simulink model "MOBATSim"  (R2020b)
settings: Solver=FixedStepAuto  StartTime=0.0  StopTime=Sim_t  FixedStep=0.01  MinStep=0.01  RelTol=1e-2
values from neighbouring files (symbols this model uses):
  maxSpeed = car.dynamics.maxSpeed    [VehiclePathPlanner.m]    (also in VehiclePathPlanner1.m; VehiclePathPlanner_AStar.m; VehiclePathPlanner_Astar.m; VehiclePathPlanner_DStarExtraLight.m)
  Vehicles = evalin('base','Vehicles')    [Infrastructure.m]    (also in VehicleSensors.m)
undefined symbols (not defined in the file or in its folder): default_spacing, delayTimeV3, FI_distance, FI_speed, max_ac, meters, min_ac, MinDeceleration, SafeDistance, Sim_Ts, time_gap, Ts, v_set, Vehicle_id, verr_gain, vx_gain, xerr_gain
libraries: simulink x43, pid_lib x15, drivingvehiclecontroller x11, robotmobilelib x11, autolibshared x4, robotalgslib x3, mpcadaslib x1
(part 2 of 7)

== system MOBATSim/Vehicle Model 6 ==
  note: Perception
  note: Decision-Making
  note: Control
  Behavioural Planner : MATLABSystem  System=VehicleDrivingMode  Vehicle_id=Vehicle_id  SimulateUsing=Interpreted execution
      mask Type: VehicleDrivingMode
      mask Display:
      | image('BehaviouralPlanner.png');
      | port_label('input',1,'LeaderSpeed');
      | port_label('input',2,'LeaderDistance');
      | port_label('input',3,'emergencyCase');
      | port_label('output',1,'SpeedReference');
      | port_label('output',2,'DistanceReference');
      | port_label('output',3,'LeadSpeed');
      | port_label('output',4,'DrivingMode');
      | port_label('output',5,'Dist2Stop');
      | port_label('output',6,'laneChange');
  Longitudinal and Lateral Controllers : Subsystem
  Safety Filter : Subsystem
  Transform to MOBATSim Coordinates : Subsystem
  Vehicle Model - Kinematic 3DOF Single Track : Subsystem  mask{Vehicle_id=Vehicle_id}
      mask prompts: Vehicle_id "Vehicle ID"
  Vehicle Path Planner : MATLABSystem  System=VehiclePathPlanner_Astar  Vehicle_id=Vehicle_id  SimulateUsing=Interpreted execution
      mask Type: VehiclePathPlanner_Astar
      mask Display:
      | image('PathPlanner.png');
      | port_label('input',1,'CommunicationIDs');
      | port_label('output',1,'waypointReached');
  Vehicle Sensors : MATLABSystem  System=VehicleSensors  Vehicle_id=Vehicle_id  Tsample=Sim_Ts  OffsetTime=0  SimulateUsing=Interpreted execution
      mask Type: VehicleSensors
      mask Display:
      | image('sensor.png');
      | port_label('output',1,'V2VcommIDs');
      | port_label('output',2,'distanceToLeading');
  Vehicle Situation Awareness : MATLABSystem  System=VehicleSituationAwareness  Vehicle_id=Vehicle_id  SimulateUsing=Interpreted execution
      mask Type: VehicleSituationAwareness
      mask Display:
      | image('situationAwareness.png');
      | port_label('input',1,'detectionFrontSensor');
      | port_label('output',1,'leaderSpeed');
      | port_label('output',2,'leaderDistance');
      | port_label('output',3,'emergencyCase');
  Vehicle V2I Output : MATLABSystem  System=VehicleV2I_Out  Vehicle_id=Vehicle_id  SimulateUsing=Interpreted execution
      mask Type: VehicleV2I_Out
      mask Display:
      | image('V2I.png');
      | port_label('input',1,'waypointReached');
      | port_label('output',1,'V2Idata');
  Position : Outport  VectorParamsAs1DForOutWhenUnconnected=off
  Orientation : Outport  Port=2  VectorParamsAs1DForOutWhenUnconnected=off
  Speed : Outport  Port=3  VectorParamsAs1DForOutWhenUnconnected=off
  V_Network_Out : Outport  Port=4  VectorParamsAs1DForOutWhenUnconnected=off
  wires:
  Vehicle Sensors/2 -> Vehicle Situation Awareness/1
  Vehicle Situation Awareness/1 -> Behavioural Planner/1
  Vehicle Path Planner/1 -> Vehicle V2I Output/1
  Vehicle Sensors/1 -> Vehicle Path Planner/1
  Vehicle V2I Output/1 -> V_Network_Out/1
  Vehicle Situation Awareness/3 -> Behavioural Planner/3
  Vehicle Situation Awareness/2 -> Behavioural Planner/2
  Behavioural Planner/1 -> Longitudinal and Lateral Controllers/1(Speed Reference)
  Behavioural Planner/2 -> Longitudinal and Lateral Controllers/2(Inter Vehicular Distance)
  Behavioural Planner/3 -> Longitudinal and Lateral Controllers/3(Lead Speed)
  Behavioural Planner/4 -> Longitudinal and Lateral Controllers/4(drivingMode)
  Behavioural Planner/5 -> Longitudinal and Lateral Controllers/5(Dist2Stop)
  Transform to MOBATSim Coordinates/1(Position) -> Position/1
  Transform to MOBATSim Coordinates/2(Orientation) -> Orientation/1
  Vehicle Model - Kinematic 3DOF Single Track/2(xdot) -> Longitudinal and Lateral Controllers/7(Actual Speed), Speed/1
  Vehicle Model - Kinematic 3DOF Single Track/1(Pose) -> Longitudinal and Lateral Controllers/8(Actual Pose), Transform to MOBATSim Coordinates/1(Pose)
  Longitudinal and Lateral Controllers/1(ref Acc) -> Safety Filter/1(Reference Acceleration)
  Longitudinal and Lateral Controllers/2(ref Steering) -> Safety Filter/2(Reference Steering Angle)
  Safety Filter/1(Steering Angle Cmd) -> Vehicle Model - Kinematic 3DOF Single Track/1(WhlAngF)
  Safety Filter/2(Speed_input) -> Vehicle Model - Kinematic 3DOF Single Track/2(xdotin)
  Behavioural Planner/6 -> Longitudinal and Lateral Controllers/6(laneChange)

== system MOBATSim/Vehicle Model 7 ==
  note: Perception
  note: Decision-Making
  note: Control
  Behavioural Planner : MATLABSystem  System=VehicleDrivingMode  Vehicle_id=Vehicle_id  SimulateUsing=Interpreted execution
      mask Type: VehicleDrivingMode
      mask Display:
      | image('BehaviouralPlanner.png');
      | port_label('input',1,'LeaderSpeed');
      | port_label('input',2,'LeaderDistance');
      | port_label('input',3,'emergencyCase');
      | port_label('output',1,'SpeedReference');
      | port_label('output',2,'DistanceReference');
      | port_label('output',3,'LeadSpeed');
      | port_label('output',4,'DrivingMode');
      | port_label('output',5,'Dist2Stop');
      | port_label('output',6,'laneChange');
  Longitudinal and Lateral Controllers : Subsystem
  Safety Filter : Subsystem
  Transform to MOBATSim Coordinates : Subsystem
  Vehicle Model - Kinematic 3DOF Single Track : Subsystem  mask{Vehicle_id=Vehicle_id}
      mask prompts: Vehicle_id "Vehicle ID"
  Vehicle Path Planner : MATLABSystem  System=VehiclePathPlanner_Astar  Vehicle_id=Vehicle_id  SimulateUsing=Interpreted execution
      mask Type: VehiclePathPlanner_Astar
      mask Display:
      | image('PathPlanner.png');
      | port_label('input',1,'CommunicationIDs');
      | port_label('output',1,'waypointReached');
  Vehicle Sensors : MATLABSystem  System=VehicleSensors  Vehicle_id=Vehicle_id  Tsample=Sim_Ts  OffsetTime=0  SimulateUsing=Interpreted execution
      mask Type: VehicleSensors
      mask Display:
      | image('sensor.png');
      | port_label('output',1,'V2VcommIDs');
      | port_label('output',2,'distanceToLeading');
  Vehicle Situation Awareness : MATLABSystem  System=VehicleSituationAwareness  Vehicle_id=Vehicle_id  SimulateUsing=Interpreted execution
      mask Type: VehicleSituationAwareness
      mask Display:
      | image('situationAwareness.png');
      | port_label('input',1,'detectionFrontSensor');
      | port_label('output',1,'leaderSpeed');
      | port_label('output',2,'leaderDistance');
      | port_label('output',3,'emergencyCase');
  Vehicle V2I Output : MATLABSystem  System=VehicleV2I_Out  Vehicle_id=Vehicle_id  SimulateUsing=Interpreted execution
      mask Type: VehicleV2I_Out
      mask Display:
      | image('V2I.png');
      | port_label('input',1,'waypointReached');
      | port_label('output',1,'V2Idata');
  Position : Outport  VectorParamsAs1DForOutWhenUnconnected=off
  Orientation : Outport  Port=2  VectorParamsAs1DForOutWhenUnconnected=off
  Speed : Outport  Port=3  VectorParamsAs1DForOutWhenUnconnected=off
  V_Network_Out : Outport  Port=4  VectorParamsAs1DForOutWhenUnconnected=off
  wires:
  Vehicle Sensors/2 -> Vehicle Situation Awareness/1
  Vehicle Situation Awareness/1 -> Behavioural Planner/1
  Vehicle Path Planner/1 -> Vehicle V2I Output/1
  Vehicle Sensors/1 -> Vehicle Path Planner/1
  Vehicle V2I Output/1 -> V_Network_Out/1
  Vehicle Situation Awareness/3 -> Behavioural Planner/3
  Vehicle Situation Awareness/2 -> Behavioural Planner/2
  Behavioural Planner/1 -> Longitudinal and Lateral Controllers/1(Speed Reference)
  Behavioural Planner/2 -> Longitudinal and Lateral Controllers/2(Inter Vehicular Distance)
  Behavioural Planner/3 -> Longitudinal and Lateral Controllers/3(Lead Speed)
  Behavioural Planner/4 -> Longitudinal and Lateral Controllers/4(drivingMode)
  Behavioural Planner/5 -> Longitudinal and Lateral Controllers/5(Dist2Stop)
  Transform to MOBATSim Coordinates/1(Position) -> Position/1
  Transform to MOBATSim Coordinates/2(Orientation) -> Orientation/1
  Vehicle Model - Kinematic 3DOF Single Track/2(xdot) -> Longitudinal and Lateral Controllers/7(Actual Speed), Speed/1
  Vehicle Model - Kinematic 3DOF Single Track/1(Pose) -> Longitudinal and Lateral Controllers/8(Actual Pose), Transform to MOBATSim Coordinates/1(Pose)
  Longitudinal and Lateral Controllers/1(ref Acc) -> Safety Filter/1(Reference Acceleration)
  Longitudinal and Lateral Controllers/2(ref Steering) -> Safety Filter/2(Reference Steering Angle)
  Safety Filter/1(Steering Angle Cmd) -> Vehicle Model - Kinematic 3DOF Single Track/1(WhlAngF)
  Safety Filter/2(Speed_input) -> Vehicle Model - Kinematic 3DOF Single Track/2(xdotin)
  Behavioural Planner/6 -> Longitudinal and Lateral Controllers/6(laneChange)

== system MOBATSim/Vehicle Model 8 ==
  note: Perception
  note: Decision-Making
  note: Control
  Behavioural Planner : MATLABSystem  System=VehicleDrivingMode  Vehicle_id=Vehicle_id  SimulateUsing=Interpreted execution
      mask Type: VehicleDrivingMode
      mask Display:
      | image('BehaviouralPlanner.png');
      | port_label('input',1,'LeaderSpeed');
      | port_label('input',2,'LeaderDistance');
      | port_label('input',3,'emergencyCase');
      | port_label('output',1,'SpeedReference');
      | port_label('output',2,'DistanceReference');
      | port_label('output',3,'LeadSpeed');
      | port_label('output',4,'DrivingMode');
      | port_label('output',5,'Dist2Stop');
      | port_label('output',6,'laneChange');
  Longitudinal and Lateral Controllers : Subsystem
  Safety Filter : Subsystem
  Transform to MOBATSim Coordinates : Subsystem
  Vehicle Model - Kinematic 3DOF Single Track : Subsystem  mask{Vehicle_id=Vehicle_id}
      mask prompts: Vehicle_id "Vehicle ID"
  Vehicle Path Planner : MATLABSystem  System=VehiclePathPlanner_Astar  Vehicle_id=Vehicle_id  SimulateUsing=Interpreted execution
      mask Type: VehiclePathPlanner_Astar
      mask Display:
      | image('PathPlanner.png');
      | port_label('input',1,'CommunicationIDs');
      | port_label('output',1,'waypointReached');
  Vehicle Sensors : MATLABSystem  System=VehicleSensors  Vehicle_id=Vehicle_id  Tsample=Sim_Ts  OffsetTime=0  SimulateUsing=Interpreted execution
      mask Type: VehicleSensors
      mask Display:
      | image('sensor.png');
      | port_label('output',1,'V2VcommIDs');
      | port_label('output',2,'distanceToLeading');
  Vehicle Situation Awareness : MATLABSystem  System=VehicleSituationAwareness  Vehicle_id=Vehicle_id  SimulateUsing=Interpreted execution
      mask Type: VehicleSituationAwareness
      mask Display:
      | image('situationAwareness.png');
      | port_label('input',1,'detectionFrontSensor');
      | port_label('output',1,'leaderSpeed');
      | port_label('output',2,'leaderDistance');
      | port_label('output',3,'emergencyCase');
  Vehicle V2I Output : MATLABSystem  System=VehicleV2I_Out  Vehicle_id=Vehicle_id  SimulateUsing=Interpreted execution
      mask Type: VehicleV2I_Out
      mask Display:
      | image('V2I.png');
      | port_label('input',1,'waypointReached');
      | port_label('output',1,'V2Idata');
  Position : Outport  VectorParamsAs1DForOutWhenUnconnected=off
  Orientation : Outport  Port=2  VectorParamsAs1DForOutWhenUnconnected=off
  Speed : Outport  Port=3  VectorParamsAs1DForOutWhenUnconnected=off
  V_Network_Out : Outport  Port=4  VectorParamsAs1DForOutWhenUnconnected=off
  wires:
  Vehicle Sensors/2 -> Vehicle Situation Awareness/1
  Vehicle Situation Awareness/1 -> Behavioural Planner/1
  Vehicle Path Planner/1 -> Vehicle V2I Output/1
  Vehicle Sensors/1 -> Vehicle Path Planner/1
  Vehicle V2I Output/1 -> V_Network_Out/1
  Vehicle Situation Awareness/3 -> Behavioural Planner/3
  Vehicle Situation Awareness/2 -> Behavioural Planner/2
  Behavioural Planner/1 -> Longitudinal and Lateral Controllers/1(Speed Reference)
  Behavioural Planner/2 -> Longitudinal and Lateral Controllers/2(Inter Vehicular Distance)
  Behavioural Planner/3 -> Longitudinal and Lateral Controllers/3(Lead Speed)
  Behavioural Planner/4 -> Longitudinal and Lateral Controllers/4(drivingMode)
  Behavioural Planner/5 -> Longitudinal and Lateral Controllers/5(Dist2Stop)
  Transform to MOBATSim Coordinates/1(Position) -> Position/1
  Transform to MOBATSim Coordinates/2(Orientation) -> Orientation/1
  Vehicle Model - Kinematic 3DOF Single Track/2(xdot) -> Longitudinal and Lateral Controllers/7(Actual Speed), Speed/1
  Vehicle Model - Kinematic 3DOF Single Track/1(Pose) -> Longitudinal and Lateral Controllers/8(Actual Pose), Transform to MOBATSim Coordinates/1(Pose)
  Longitudinal and Lateral Controllers/1(ref Acc) -> Safety Filter/1(Reference Acceleration)
  Longitudinal and Lateral Controllers/2(ref Steering) -> Safety Filter/2(Reference Steering Angle)
  Safety Filter/1(Steering Angle Cmd) -> Vehicle Model - Kinematic 3DOF Single Track/1(WhlAngF)
  Safety Filter/2(Speed_input) -> Vehicle Model - Kinematic 3DOF Single Track/2(xdotin)
  Behavioural Planner/6 -> Longitudinal and Lateral Controllers/6(laneChange)

== system MOBATSim/Vehicle Model 9 ==
  note: Perception
  note: Decision-Making
  note: Control
  Behavioural Planner : MATLABSystem  System=VehicleDrivingMode  Vehicle_id=Vehicle_id  SimulateUsing=Interpreted execution
      mask Type: VehicleDrivingMode
      mask Display:
      | image('BehaviouralPlanner.png');
      | port_label('input',1,'LeaderSpeed');
      | port_label('input',2,'LeaderDistance');
      | port_label('input',3,'emergencyCase');
      | port_label('output',1,'SpeedReference');
      | port_label('output',2,'DistanceReference');
      | port_label('output',3,'LeadSpeed');
      | port_label('output',4,'DrivingMode');
      | port_label('output',5,'Dist2Stop');
      | port_label('output',6,'laneChange');
  Longitudinal and Lateral Controllers : Subsystem
  Safety Filter : Subsystem
  Transform to MOBATSim Coordinates : Subsystem
  Vehicle Model - Kinematic 3DOF Single Track : Subsystem  mask{Vehicle_id=Vehicle_id}
      mask prompts: Vehicle_id "Vehicle ID"
  Vehicle Path Planner : MATLABSystem  System=VehiclePathPlanner_Astar  Vehicle_id=Vehicle_id  SimulateUsing=Interpreted execution
      mask Type: VehiclePathPlanner_Astar
      mask Display:
      | image('PathPlanner.png');
      | port_label('input',1,'CommunicationIDs');
      | port_label('output',1,'waypointReached');
  Vehicle Sensors : MATLABSystem  System=VehicleSensors  Vehicle_id=Vehicle_id  Tsample=Sim_Ts  OffsetTime=0  SimulateUsing=Interpreted execution
      mask Type: VehicleSensors
      mask Display:
      | image('sensor.png');
      | port_label('output',1,'V2VcommIDs');
      | port_label('output',2,'distanceToLeading');
  Vehicle Situation Awareness : MATLABSystem  System=VehicleSituationAwareness  Vehicle_id=Vehicle_id  SimulateUsing=Interpreted execution
      mask Type: VehicleSituationAwareness
      mask Display:
      | image('situationAwareness.png');
      | port_label('input',1,'detectionFrontSensor');
      | port_label('output',1,'leaderSpeed');
      | port_label('output',2,'leaderDistance');
      | port_label('output',3,'emergencyCase');
  Vehicle V2I Output : MATLABSystem  System=VehicleV2I_Out  Vehicle_id=Vehicle_id  SimulateUsing=Interpreted execution
      mask Type: VehicleV2I_Out
      mask Display:
      | image('V2I.png');
      | port_label('input',1,'waypointReached');
      | port_label('output',1,'V2Idata');
  Position : Outport  VectorParamsAs1DForOutWhenUnconnected=off
  Orientation : Outport  Port=2  VectorParamsAs1DForOutWhenUnconnected=off
  Speed : Outport  Port=3  VectorParamsAs1DForOutWhenUnconnected=off
  V_Network_Out : Outport  Port=4  VectorParamsAs1DForOutWhenUnconnected=off
  wires:
  Vehicle Sensors/2 -> Vehicle Situation Awareness/1
  Vehicle Situation Awareness/1 -> Behavioural Planner/1
  Vehicle Path Planner/1 -> Vehicle V2I Output/1
  Vehicle Sensors/1 -> Vehicle Path Planner/1
  Vehicle V2I Output/1 -> V_Network_Out/1
  Vehicle Situation Awareness/3 -> Behavioural Planner/3
  Vehicle Situation Awareness/2 -> Behavioural Planner/2
  Behavioural Planner/1 -> Longitudinal and Lateral Controllers/1(Speed Reference)
  Behavioural Planner/2 -> Longitudinal and Lateral Controllers/2(Inter Vehicular Distance)
  Behavioural Planner/3 -> Longitudinal and Lateral Controllers/3(Lead Speed)
  Behavioural Planner/4 -> Longitudinal and Lateral Controllers/4(drivingMode)
  Behavioural Planner/5 -> Longitudinal and Lateral Controllers/5(Dist2Stop)
  Transform to MOBATSim Coordinates/1(Position) -> Position/1
  Transform to MOBATSim Coordinates/2(Orientation) -> Orientation/1
  Vehicle Model - Kinematic 3DOF Single Track/2(xdot) -> Longitudinal and Lateral Controllers/7(Actual Speed), Speed/1
  Vehicle Model - Kinematic 3DOF Single Track/1(Pose) -> Longitudinal and Lateral Controllers/8(Actual Pose), Transform to MOBATSim Coordinates/1(Pose)
  Longitudinal and Lateral Controllers/1(ref Acc) -> Safety Filter/1(Reference Acceleration)
  Longitudinal and Lateral Controllers/2(ref Steering) -> Safety Filter/2(Reference Steering Angle)
  Safety Filter/1(Steering Angle Cmd) -> Vehicle Model - Kinematic 3DOF Single Track/1(WhlAngF)
  Safety Filter/2(Speed_input) -> Vehicle Model - Kinematic 3DOF Single Track/2(xdotin)
  Behavioural Planner/6 -> Longitudinal and Lateral Controllers/6(laneChange)

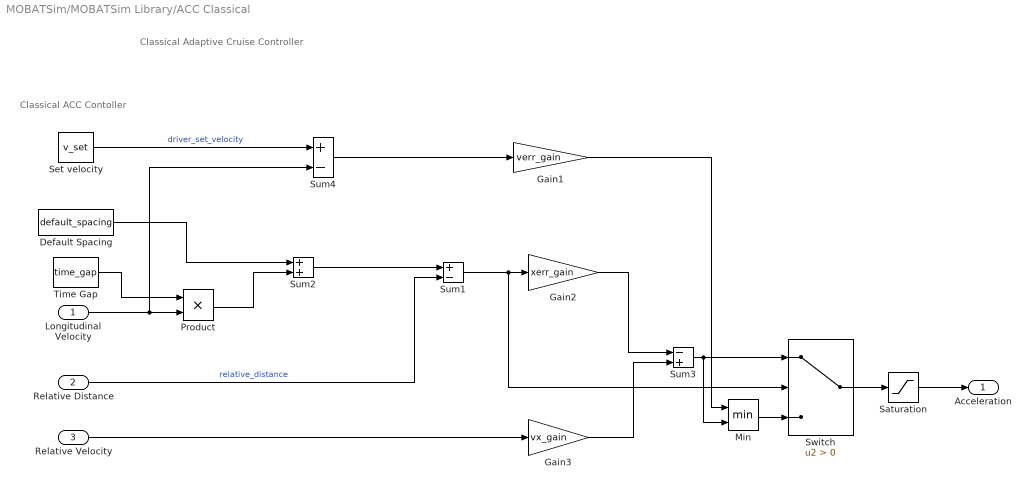
== system MOBATSim/MOBATSim Library/ACC Classical ==
  note: Classical ACC Contoller
  note: Classical Adaptive Cruise Controller
  Longitudinal Velocity : Inport
  Relative Distance : Inport  Port=2
  Relative Velocity : Inport  Port=3
  Default Spacing : Constant  Value=default_spacing  SampleTime=Ts
  Gain1 : Gain  Gain=verr_gain
  Gain2 : Gain  Gain=xerr_gain
  Gain3 : Gain  Gain=vx_gain
  Min : MinMax  Inputs=2
  Product : Product
  Saturation : Saturate  UpperLimit=max_ac  LowerLimit=min_ac
  Set velocity : Constant  Value=v_set  SampleTime=Ts
  Sum1 : Sum  Inputs=+-
  Sum2 : Sum
  Sum3 : Sum  Inputs=-+
  Sum4 : Sum  Inputs=+-
  Switch : Switch  Criteria=u2 > Threshold
  Time Gap : Constant  Value=time_gap  SampleTime=Ts
  Acceleration : Outport  VectorParamsAs1DForOutWhenUnconnected=off
  wires:
  Longitudinal Velocity/1 -> Product/2, Sum4/2
  Default Spacing/1 -> Sum2/1
  Gain2/1 -> Sum3/1
  Sum4/1 -> Gain1/1
  Min/1 -> Switch/3
  Gain3/1 -> Sum3/2
  Switch/1 -> Saturation/1
  Relative Velocity/1 -> Gain3/1
  Time Gap/1 -> Product/1
  Saturation/1 -> Acceleration/1
  Product/1 -> Sum2/2
  Set velocity/1 -> Sum4/1  "driver_set_velocity"
  Sum3/1 -> Min/2, Switch/1
  Sum1/1 -> Switch/2, Gain2/1
  Gain1/1 -> Min/1
  Relative Distance/1 -> Sum1/2  "relative_distance"
  Sum2/1 -> Sum1/1

== system MOBATSim/MOBATSim Library/Old Vehicle 3 Dynamic Bicycle Model with Pure Pursuit ==
  Speed Reference : Inport
  Inter Vehicular Distance : Inport  Port=2
  Lead Speed : Inport  Port=3
  drivingMode : Inport  Port=4
  CollisionStatus : Inport  Port=5
  Dist2Stop : Inport  Port=6
  Longitudinal Speed Control : Subsystem
  Reference Waypoint Generation : Subsystem
  Vehicle Dynamics Interface : Subsystem
  Vehicle Kinematic 3DOF Single Track : Subsystem  mask{Vehicle_id=Vehicle_id}
      mask prompts: Vehicle_id "Vehicle ID"
  X : Outport
  Y : Outport  Port=2
  yaw : Outport  Port=3
  wires:
  Reference Waypoint Generation/1(Target Direction) -> Vehicle Dynamics Interface/3(Target Direction)
  Vehicle Kinematic 3DOF Single Track/4(xdot) -> Longitudinal Speed Control/6(Actual Speed), Reference Waypoint Generation/4(Speed)
  Lead Speed/1 -> Longitudinal Speed Control/3(Lead Speed)
  Vehicle Dynamics Interface/1(Actual Steering Angle) -> Vehicle Kinematic 3DOF Single Track/1(WhlAngF)
  CollisionStatus/1 -> Vehicle Dynamics Interface/2(CollisionStatus)
  Vehicle Kinematic 3DOF Single Track/1(X) -> X/1, Reference Waypoint Generation/1(Xpos)
  Dist2Stop/1 -> Longitudinal Speed Control/5(Dist2Stop)
  Vehicle Dynamics Interface/2(Actual Speed) -> Vehicle Kinematic 3DOF Single Track/2(xdotin)
  drivingMode/1 -> Longitudinal Speed Control/4(Driving Mode), Reference Waypoint Generation/5(drivingMode)
  Vehicle Kinematic 3DOF Single Track/2(Y) -> Y/1, Reference Waypoint Generation/2(Ypos)
  Vehicle Kinematic 3DOF Single Track/3(yaw) -> yaw/1, Reference Waypoint Generation/3(Psi)
  Longitudinal Speed Control/1(Longitduinal Acceleration Command) -> Vehicle Dynamics Interface/1(Acceleration)
  Speed Reference/1 -> Longitudinal Speed Control/1(Speed Reference)
  Inter Vehicular Distance/1 -> Longitudinal Speed Control/2(Inter Vehicular Distance)

== system MOBATSim/MOBATSim Library/Old Vehicle 5 Dual Track ==
  Speed Reference : Inport
  Inter Vehicular Distance : Inport  Port=2
  Lead Speed : Inport  Port=3
  drivingMode : Inport  Port=4
  CollisionStatus : Inport  Port=5
  Dist2Stop : Inport  Port=6
  Longitudinal Speed Control : Subsystem
  Reference Waypoint Generation : Subsystem
  Vehicle Dynamics Interface : Subsystem
  Vehicle Kinematic 3DOF Single Track : Subsystem  mask{Vehicle_id=Vehicle_id}
      mask prompts: Vehicle_id "Vehicle ID"
  X : Outport
  Y : Outport  Port=2
  yaw : Outport  Port=3
  wires:
  Vehicle Kinematic 3DOF Single Track/1(X) -> X/1, Reference Waypoint Generation/1(Xpos)
  Reference Waypoint Generation/1(SteerCmd_Stanley) -> Vehicle Dynamics Interface/3(SteerCmd_Stanley)
  Vehicle Dynamics Interface/2(Actual Speed) -> Vehicle Kinematic 3DOF Single Track/2(xdotin)
  Vehicle Kinematic 3DOF Single Track/2(Y) -> Y/1, Reference Waypoint Generation/2(Ypos)
  Vehicle Kinematic 3DOF Single Track/4(xdot) -> Longitudinal Speed Control/6(Actual Speed), Reference Waypoint Generation/4(Speed)
  drivingMode/1 -> Reference Waypoint Generation/5(drivingMode), Longitudinal Speed Control/4(Driving Mode)
  Vehicle Dynamics Interface/1(Actual Steering Angle) -> Vehicle Kinematic 3DOF Single Track/1(WhlAngF)
  Vehicle Kinematic 3DOF Single Track/3(yaw) -> yaw/1, Reference Waypoint Generation/3(Psi)
  Longitudinal Speed Control/1(Longitduinal Acceleration Command) -> Vehicle Dynamics Interface/1(Acceleration)
  Dist2Stop/1 -> Longitudinal Speed Control/5(Dist2Stop)
  CollisionStatus/1 -> Vehicle Dynamics Interface/2(CollisionStatus)
  Inter Vehicular Distance/1 -> Longitudinal Speed Control/2(Inter Vehicular Distance)
  Lead Speed/1 -> Longitudinal Speed Control/3(Lead Speed)
  Speed Reference/1 -> Longitudinal Speed Control/1(Speed Reference)

== system MOBATSim/MOBATSim Library/Platoon Controller - PID ==
  Inter Vehicular Distance : Inport
  Lead Speed : Inport  Port=2
  Vehicle Speed : Inport  Port=3
  Compare To Constant : simulink/Logic and Bit Operations/Compare To Constant  relop=>  const=2  OutDataTypeStr=uint8
  Constant : Constant  Value=meters
  Gain : Gain  Gain=1.4
  Multiport Switch : MultiPortSwitch  DataPortOrder=Zero-based contiguous  Inputs=2  zeroidx=on
  PID Controller5 : pid_lib/PID Controller  Controller=PID  Form=Parallel  TimeDomain=Continuous-time  UseExternalTs=off  SampleTime=-1  IntegratorMethod=Forward Euler  FilterMethod=Forward Euler  ControllerParametersSource=internal  P=2.0341199375219  I=0.0356576460366845  D=2.08363010404189  UseFilter=on  N=233.214579742572  TunerSelectOption=Transfer Function Based (PID Tuner App)  InitialConditionSource=internal  InitialConditionForIntegrator=0  InitialConditionForFilter=0  DifferentiatorICPrevScaledInput=0  ExternalReset=none  TrackingMode=off  Kt=1  LimitOutput=on  SatLimitsSource=internal  UpperSaturationLimit=100  LowerSaturationLimit=-100  LinearizeAsGain=on  AntiWindupMode=clamping  Kb=1  POutMin=[]  POutMax=[]  IOutMin=[]  IOutMax=[]  DOutMin=[]  DOutMax=[]  NOutMin=[]  NOutMax=[]  SumOutMin=[]  SumOutMax=[]  SaturationOutMin=[]  SaturationOutMax=[]  PParamMin=[]  PParamMax=[]  IParamMin=[]  IParamMax=[]  DParamMin=[]  DParamMax=[]  NParamMin=[]  NParamMax=[]  KbParamMin=[]  KbParamMax=[]  KtParamMin=[]  KtParamMax=[]  KbOutMin=[]  KbOutMax=[]  KtOutMin=[]  KtOutMax=[]  IntegratorOutMin=[]  IntegratorOutMax=[]  FilterOutMin=[]  FilterOutMax=[]  SumI1OutMin=[]  SumI1OutMax=[]  SumI2OutMin=[]  SumI2OutMax=[]  SumI3OutMin=[]  SumI3OutMax=[]  SumI4OutMin=[]  SumI4OutMax=[]  SumDOutMin=[]  SumDOutMax=[]  DifferentiatorOutMin=[]  DifferentiatorOutMax=[]  FilterDiffOutCoefMin=[]  FilterDiffOutCoefMax=[]  ReciprocalOutMin=[]  ReciprocalOutMax=[]  SumDenOutMin=[]  SumDenOutMax=[]  SumNumOutMin=[]  SumNumOutMax=[]  DivideOutMin=[]  DivideOutMax=[]  UdiffTsProdOutMin=[]  UdiffTsProdOutMax=[]  NTsProdOutMin=[]  NTsProdOutMax=[]  UintegralTsProdOutMin=[]  UintegralTsProdOutMax=[]  UngainTsProdOutMin=[]  UngainTsProdOutMax=[]  IntegratorContinuousStateAttributes=''  IntegratorStateMustResolveToSignalObject=off  IntegratorRTWStateStorageClass=Auto  FilterContinuousStateAttributes=''  FilterStateMustResolveToSignalObject=off  FilterRTWStateStorageClass=Auto  ParallelPVariant=InternalParameters  IdealPVariant=Disabled  IVariant=InternalParameters  DVariant=InternalParameters  IntegratorVariant=Continuous  SatVariant=Enabled  AWVariant=ContClampingParallel  PCopyVariant=Disabled  TRVariant=Disabled  FdbkBlocksVariant=Forward  IdealPFdbkVariant=Disabled  SatFdbkVariant=Disabled  DerivativeFilterVariant=ContFilter  NVariant=InternalParameters  NCopyVariant=Disabled  FilterICVariant=InternalICsFilter  IntegratorICVariant=InternalICs  ExternalResetVariant=Disabled  TRSumVariant=Passthrough  SumFdbkVariant=Disabled  SumVariant=Sum_PID  TsampFilterVariant=InternalTs  TsampNgainVariant=Passthrough  TsampIntegralVariant=Passthrough  ExternalSaturationOutDataTypeStr=Inherit: Same as second input
  Sum : Sum  Inputs=|-+
  Sum1 : Sum  Inputs=|++
  Sum2 : Sum  Inputs=|+-
  Transfer Fcn : TransferFcn  Numerator=[0.05]  Denominator=[1 2]
  ref speed : Outport  VectorParamsAs1DForOutWhenUnconnected=off
  wires:
  Transfer Fcn/1 -> PID Controller5/1
  Vehicle Speed/1 -> Gain/1, Sum/1
  PID Controller5/1 -> Multiport Switch/2
  Sum/1 -> Compare To Constant/1
  Multiport Switch/1 -> ref speed/1
  Compare To Constant/1 -> Multiport Switch/1
  Lead Speed/1 -> Sum/2, Multiport Switch/3
  Constant/1 -> Sum1/1
  Sum1/1 -> Sum2/2
  Gain/1 -> Sum1/2
  Sum2/1 -> Transfer Fcn/1
  Inter Vehicular Distance/1 -> Sum2/1

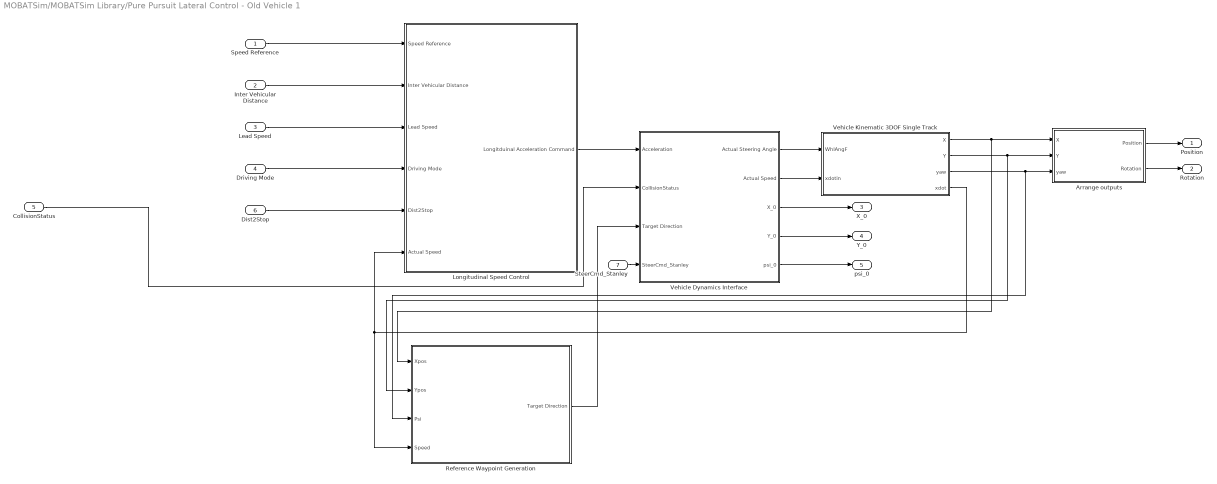
== system MOBATSim/MOBATSim Library/Pure Pursuit Lateral Control - Old Vehicle 1 ==
  Speed Reference : Inport
  Inter Vehicular Distance : Inport  Port=2
  Lead Speed : Inport  Port=3
  Driving Mode : Inport  Port=4
  CollisionStatus : Inport  Port=5
  Dist2Stop : Inport  Port=6
  SteerCmd_Stanley : Inport  Port=7
  Arrange outputs : Subsystem
  Longitudinal Speed Control : Subsystem
  Reference Waypoint Generation : Subsystem
  Vehicle Dynamics Interface : Subsystem
  Vehicle Kinematic 3DOF Single Track : Subsystem  mask{Vehicle_id=Vehicle_id}
      mask prompts: Vehicle_id "Vehicle ID"
  Position : Outport
  Rotation : Outport  Port=2
  X_0 : Outport  Port=3
  Y_0 : Outport  Port=4
  psi_0 : Outport  Port=5
  wires:
  Reference Waypoint Generation/1(Target Direction) -> Vehicle Dynamics Interface/3(Target Direction)
  Vehicle Kinematic 3DOF Single Track/1(X) -> Reference Waypoint Generation/1(Xpos), Arrange outputs/1(X)
  Vehicle Kinematic 3DOF Single Track/4(xdot) -> Longitudinal Speed Control/6(Actual Speed), Reference Waypoint Generation/4(Speed)
  SteerCmd_Stanley/1 -> Vehicle Dynamics Interface/4(SteerCmd_Stanley)
  Vehicle Dynamics Interface/2(Actual Speed) -> Vehicle Kinematic 3DOF Single Track/2(xdotin)
  Vehicle Dynamics Interface/1(Actual Steering Angle) -> Vehicle Kinematic 3DOF Single Track/1(WhlAngF)
  Vehicle Kinematic 3DOF Single Track/3(yaw) -> Reference Waypoint Generation/3(Psi), Arrange outputs/3(yaw)
  Longitudinal Speed Control/1(Longitduinal Acceleration Command) -> Vehicle Dynamics Interface/1(Acceleration)
  Vehicle Kinematic 3DOF Single Track/2(Y) -> Arrange outputs/2(Y), Reference Waypoint Generation/2(Ypos)
  Arrange outputs/1(Position) -> Position/1
  Inter Vehicular Distance/1 -> Longitudinal Speed Control/2(Inter Vehicular Distance)
  Driving Mode/1 -> Longitudinal Speed Control/4(Driving Mode)
  Dist2Stop/1 -> Longitudinal Speed Control/5(Dist2Stop)
  Lead Speed/1 -> Longitudinal Speed Control/3(Lead Speed)
  Speed Reference/1 -> Longitudinal Speed Control/1(Speed Reference)
  CollisionStatus/1 -> Vehicle Dynamics Interface/2(CollisionStatus)
  Vehicle Dynamics Interface/4(Y_0) -> Y_0/1
  Vehicle Dynamics Interface/3(X_0) -> X_0/1
  Arrange outputs/2(Rotation) -> Rotation/1
  Vehicle Dynamics Interface/5(psi_0) -> psi_0/1

== system MOBATSim/MOBATSim Library/Vehicle Model 5x ==
  note: Trajectory Planner
  note: Perception
  note: Decision Making
  Arrange outputs : Subsystem
  Behavioural Planner : MATLABSystem  System=VehicleDrivingMode  Vehicle_id=Vehicle_id  SimulateUsing=Interpreted execution
      mask Type: VehicleDrivingMode
      mask Display:
      | image('BehaviouralPlanner.png');
      | port_label('input',1,'LeaderSpeed');
      | port_label('input',2,'LeaderDistance');
      | port_label('input',3,'emergencyCase');
      | port_label('output',1,'SpeedReference');
      | port_label('output',2,'DistanceReference');
      | port_label('output',3,'LeadSpeed');
      | port_label('output',4,'DrivingMode');
      | port_label('output',5,'Dist2Stop');
  Old Vehicle 5 Dual Track : Subsystem
  Vehicle Path Planner : MATLABSystem  System=VehiclePathPlanner_Astar  Vehicle_id=Vehicle_id  SimulateUsing=Interpreted execution
      mask Type: VehiclePathPlanner_Astar
      mask Display:
      | image('PathPlanner.png');
      | port_label('input',1,'CommunicationIDs');
      | port_label('output',1,'waypointReached');
  Vehicle Sensors : MATLABSystem  System=VehicleSensors  Vehicle_id=Vehicle_id  Tsample=Sim_Ts  OffsetTime=0  SimulateUsing=Interpreted execution
      mask Type: VehicleSensors
      mask Display:
      | image('sensor.png');
      | port_label('output',1,'V2VcommIDs');
      | port_label('output',2,'distanceToLeading');
  Vehicle Situation Awareness : MATLABSystem  System=VehicleSituationAwareness  Vehicle_id=Vehicle_id  SimulateUsing=Interpreted execution
      mask Type: VehicleSituationAwareness
      mask Display:
      | image('situationAwareness.png');
      | port_label('input',1,'detectionFrontSensor');
      | port_label('output',1,'leaderSpeed');
      | port_label('output',2,'leaderDistance');
      | port_label('output',3,'emergencyCase');
  Vehicle V2I Output : MATLABSystem  System=VehicleV2I_Out  Vehicle_id=Vehicle_id  SimulateUsing=Interpreted execution
      mask Type: VehicleV2I_Out
      mask Display:
      | image('V2I.png');
      | port_label('input',1,'waypointReached');
      | port_label('output',1,'V2Idata');
  Position : Outport  VectorParamsAs1DForOutWhenUnconnected=off
  rotation : Outport  Port=2  VectorParamsAs1DForOutWhenUnconnected=off
  V_Network_Out : Outport  Port=3  VectorParamsAs1DForOutWhenUnconnected=off
  wires:
  Arrange outputs/1(Position) -> Position/1
  Arrange outputs/2(Rotation) -> rotation/1
  Vehicle Sensors/2 -> Vehicle Situation Awareness/1
  Vehicle Situation Awareness/3 -> Old Vehicle 5 Dual Track/5(CollisionStatus), Behavioural Planner/3
  Vehicle Situation Awareness/1 -> Behavioural Planner/1
  Vehicle Path Planner/1 -> Vehicle V2I Output/1
  Vehicle V2I Output/1 -> V_Network_Out/1
  Behavioural Planner/1 -> Old Vehicle 5 Dual Track/1(Speed Reference)
  Behavioural Planner/2 -> Old Vehicle 5 Dual Track/2(Inter Vehicular Distance)
  Behavioural Planner/3 -> Old Vehicle 5 Dual Track/3(Lead Speed)
  Behavioural Planner/4 -> Old Vehicle 5 Dual Track/4(drivingMode)
  Behavioural Planner/5 -> Old Vehicle 5 Dual Track/6(Dist2Stop)
  Old Vehicle 5 Dual Track/1(X) -> Arrange outputs/1(X)
  Old Vehicle 5 Dual Track/2(Y) -> Arrange outputs/2(Y)
  Old Vehicle 5 Dual Track/3(yaw) -> Arrange outputs/3(yaw)
  Vehicle Situation Awareness/2 -> Behavioural Planner/2
  Vehicle Sensors/1 -> Vehicle Path Planner/1

== system MOBATSim/Vehicle Model 1/Longitudinal and Lateral Controllers ==
  Speed Reference : Inport
  Inter Vehicular Distance : Inport  Port=2
  Lead Speed : Inport  Port=3
  drivingMode : Inport  Port=4
  Dist2Stop : Inport  Port=5
  laneChange : Inport  Port=6
  Actual Speed : Inport  Port=7
  Actual Pose : Inport  Port=8
  Lateral Control : Subsystem
  Longitudinal Speed Control : Subsystem
  ref Acc : Outport
  ref Steering : Outport  Port=2
  wires:
  laneChange/1 -> Lateral Control/3(laneChange)
  Lateral Control/1(SteerCmd_Stanley) -> ref Steering/1
  Actual Speed/1 -> Longitudinal Speed Control/6(Actual Speed), Lateral Control/1(actualSpeed)
  drivingMode/1 -> Longitudinal Speed Control/4(Driving Mode)
  Longitudinal Speed Control/1(Longitduinal Acceleration Command) -> ref Acc/1
  Dist2Stop/1 -> Longitudinal Speed Control/5(Dist2Stop)
  Inter Vehicular Distance/1 -> Longitudinal Speed Control/2(Inter Vehicular Distance)
  Lead Speed/1 -> Longitudinal Speed Control/3(Lead Speed)
  Speed Reference/1 -> Longitudinal Speed Control/1(Speed Reference)
  Actual Pose/1 -> Lateral Control/2(actualPose)

== system MOBATSim/Vehicle Model 1/Safety Filter ==
  note: Longitudinal
  Reference Acceleration : Inport
  Reference Steering Angle : Inport  Port=2
  Acceleration to Speed : Integrator  LimitOutput=on  LowerSaturationLimit=0
  MATLAB System : MATLABSystem  System=VehicleSafetyFilter  Vehicle_id=Vehicle_id  SimulateUsing=Interpreted execution
      mask Type: VehicleSafetyFilter
      mask Display:
      | disp('VehicleSafetyFilter');
      | port_label('input',1,'Acc');
      | port_label('input',2,'Steering');
      | port_label('output',1,'Acc');
      | port_label('output',2,'Stop');
      | port_label('output',3,'Steering');
  Product : Product
  Signal Specification : SignalSpecification  Dimensions=1
  Stop Check : simulink/Logic and Bit Operations/Compare To Constant  relop=~=  const=1  OutDataTypeStr=uint8
  Zero-Order Hold : ZeroOrderHold  SampleTime=Sim_Ts
  Steering Angle Cmd : Outport
  Speed_input : Outport  Port=2
  wires:
  Acceleration to Speed/1 -> Signal Specification/1
  Stop Check/1 -> Product/2
  MATLAB System/3 -> Steering Angle Cmd/1
  Signal Specification/1 -> Zero-Order Hold/1
  Reference Acceleration/1 -> MATLAB System/1
  Zero-Order Hold/1 -> Product/1
  Product/1 -> Speed_input/1
  MATLAB System/1 -> Acceleration to Speed/1
  Reference Steering Angle/1 -> MATLAB System/2
  MATLAB System/2 -> Stop Check/1

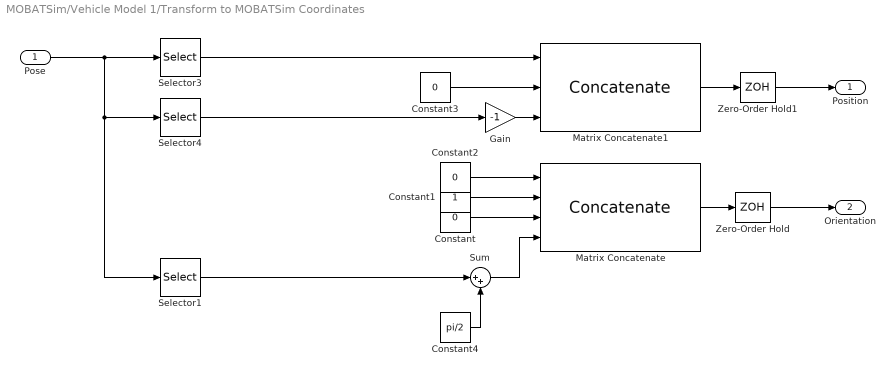
== system MOBATSim/Vehicle Model 1/Transform to MOBATSim Coordinates ==
  Pose : Inport
  Constant : Constant  Value=0
  Constant1 : Constant
  Constant2 : Constant  Value=0
  Constant3 : Constant  Value=0
  Constant4 : Constant  Value=pi/2
  Gain : Gain  Gain=-1
  Matrix Concatenate : Concatenate  NumInputs=4  ConcatenateDimension=2
  Matrix Concatenate1 : Concatenate  NumInputs=3  ConcatenateDimension=2
  Selector1 : Selector  InputPortWidth=3  IndexOptions=Index vector (dialog)  Indices=[3]  OutputSizes=1
  Selector3 : Selector  InputPortWidth=3  IndexOptions=Index vector (dialog)  Indices=[1]  OutputSizes=1
  Selector4 : Selector  InputPortWidth=3  IndexOptions=Index vector (dialog)  Indices=[2]  OutputSizes=1
  Sum : Sum  Inputs=|++
  Zero-Order Hold : ZeroOrderHold  SampleTime=Sim_Ts
  Zero-Order Hold1 : ZeroOrderHold  SampleTime=Sim_Ts
  Position : Outport
  Orientation : Outport  Port=2
  wires:
  Sum/1 -> Matrix Concatenate/4
  Constant2/1 -> Matrix Concatenate/1
  Matrix Concatenate/1 -> Zero-Order Hold/1
  Constant3/1 -> Matrix Concatenate1/2
  Gain/1 -> Matrix Concatenate1/3
  Constant4/1 -> Sum/2
  Constant1/1 -> Matrix Concatenate/2
  Matrix Concatenate1/1 -> Zero-Order Hold1/1
  Selector1/1 -> Sum/1
  Constant/1 -> Matrix Concatenate/3
  Zero-Order Hold/1 -> Orientation/1
  Zero-Order Hold1/1 -> Position/1
  Selector4/1 -> Gain/1
  Selector3/1 -> Matrix Concatenate1/1
  Pose/1 -> Selector1/1, Selector4/1, Selector3/1

== system MOBATSim/Vehicle Model 1/Vehicle Model - Kinematic 3DOF Single Track ==
  WhlAngF : Inport
  xdotin : Inport  Port=2
  Bicycle Kinematic Model : robotmobilelib/Bicycle Kinematic Model  VehicleInputs=Vehicle Speed & Steering Angle  WheelBase=3  VehicleSpeedRange=[-inf inf]  MaxSteeringAngle=pi/4  InitialState=[Vehicles(Vehicle_id).dynamics.position(1); -Vehicles(Vehicle_id).dynamics.position(3);Vehicles(Vehicle_id).dynamics.orientation(4)]  SimulateUsing=Interpreted execution
      settings: SourceProductBaseCode=RO
  Delay : Delay  DelayLength=1
  Selector3 : Selector  InputPortWidth=3  IndexOptions=Index vector (dialog)  Indices=[1]  OutputSizes=1
  Selector4 : Selector  InputPortWidth=3  IndexOptions=Index vector (dialog)  Indices=[2]  OutputSizes=1
  Sqrt : Sqrt  SaturateOnIntegerOverflow=on
  Square : Math  Operator=square  SaturateOnIntegerOverflow=on
  Square1 : Math  Operator=square  SaturateOnIntegerOverflow=on
  Sum1 : Sum  Inputs=|++
  Pose : Outport
  xdot : Outport  Port=2
  wires:
  WhlAngF/1 -> Bicycle Kinematic Model/2
  xdotin/1 -> Bicycle Kinematic Model/1
  Bicycle Kinematic Model/2 -> Selector3/1, Selector4/1
  Selector3/1 -> Square/1
  Sum1/1 -> Sqrt/1
  Square1/1 -> Sum1/2
  Selector4/1 -> Square1/1
  Sqrt/1 -> Delay/1
  Square/1 -> Sum1/1
  Delay/1 -> xdot/1
  Bicycle Kinematic Model/1 -> Pose/1

== system MOBATSim/Vehicle Model 10/Longitudinal and Lateral Controllers ==
  Speed Reference : Inport
  Inter Vehicular Distance : Inport  Port=2
  Lead Speed : Inport  Port=3
  drivingMode : Inport  Port=4
  Dist2Stop : Inport  Port=5
  laneChange : Inport  Port=6
  Actual Speed : Inport  Port=7
  Actual Pose : Inport  Port=8
  Lateral Control : Subsystem
  Longitudinal Speed Control : Subsystem
  ref Acc : Outport
  ref Steering : Outport  Port=2
  wires:
  laneChange/1 -> Lateral Control/3(laneChange)
  Lateral Control/1(SteerCmd_Stanley) -> ref Steering/1
  Actual Speed/1 -> Longitudinal Speed Control/6(Actual Speed), Lateral Control/1(actualSpeed)
  drivingMode/1 -> Longitudinal Speed Control/4(Driving Mode)
  Longitudinal Speed Control/1(Longitduinal Acceleration Command) -> ref Acc/1
  Dist2Stop/1 -> Longitudinal Speed Control/5(Dist2Stop)
  Inter Vehicular Distance/1 -> Longitudinal Speed Control/2(Inter Vehicular Distance)
  Lead Speed/1 -> Longitudinal Speed Control/3(Lead Speed)
  Speed Reference/1 -> Longitudinal Speed Control/1(Speed Reference)
  Actual Pose/1 -> Lateral Control/2(actualPose)

== system MOBATSim/Vehicle Model 10/Safety Filter ==
  note: Longitudinal
  Reference Acceleration : Inport
  Reference Steering Angle : Inport  Port=2
  Acceleration to Speed : Integrator  LimitOutput=on  LowerSaturationLimit=0
  MATLAB System : MATLABSystem  System=VehicleSafetyFilter  Vehicle_id=Vehicle_id  SimulateUsing=Interpreted execution
      mask Type: VehicleSafetyFilter
      mask Display:
      | disp('VehicleSafetyFilter');
      | port_label('input',1,'Acc');
      | port_label('input',2,'Steering');
      | port_label('output',1,'Acc');
      | port_label('output',2,'Stop');
      | port_label('output',3,'Steering');
  Product : Product
  Signal Specification : SignalSpecification  Dimensions=1
  Stop Check : simulink/Logic and Bit Operations/Compare To Constant  relop=~=  const=1  OutDataTypeStr=uint8
  Zero-Order Hold : ZeroOrderHold  SampleTime=Sim_Ts
  Steering Angle Cmd : Outport
  Speed_input : Outport  Port=2
  wires:
  Acceleration to Speed/1 -> Signal Specification/1
  Stop Check/1 -> Product/2
  MATLAB System/3 -> Steering Angle Cmd/1
  Signal Specification/1 -> Zero-Order Hold/1
  Reference Acceleration/1 -> MATLAB System/1
  Zero-Order Hold/1 -> Product/1
  Product/1 -> Speed_input/1
  MATLAB System/1 -> Acceleration to Speed/1
  Reference Steering Angle/1 -> MATLAB System/2
  MATLAB System/2 -> Stop Check/1

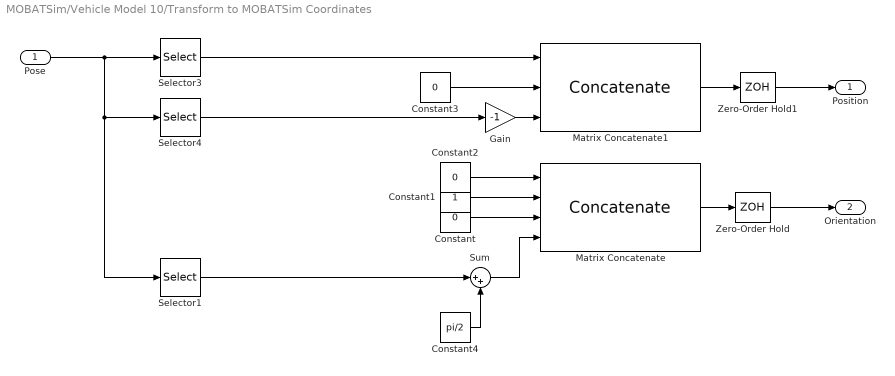
== system MOBATSim/Vehicle Model 10/Transform to MOBATSim Coordinates ==
  Pose : Inport
  Constant : Constant  Value=0
  Constant1 : Constant
  Constant2 : Constant  Value=0
  Constant3 : Constant  Value=0
  Constant4 : Constant  Value=pi/2
  Gain : Gain  Gain=-1
  Matrix Concatenate : Concatenate  NumInputs=4  ConcatenateDimension=2
  Matrix Concatenate1 : Concatenate  NumInputs=3  ConcatenateDimension=2
  Selector1 : Selector  InputPortWidth=3  IndexOptions=Index vector (dialog)  Indices=[3]  OutputSizes=1
  Selector3 : Selector  InputPortWidth=3  IndexOptions=Index vector (dialog)  Indices=[1]  OutputSizes=1
  Selector4 : Selector  InputPortWidth=3  IndexOptions=Index vector (dialog)  Indices=[2]  OutputSizes=1
  Sum : Sum  Inputs=|++
  Zero-Order Hold : ZeroOrderHold  SampleTime=Sim_Ts
  Zero-Order Hold1 : ZeroOrderHold  SampleTime=Sim_Ts
  Position : Outport
  Orientation : Outport  Port=2
  wires:
  Sum/1 -> Matrix Concatenate/4
  Constant2/1 -> Matrix Concatenate/1
  Matrix Concatenate/1 -> Zero-Order Hold/1
  Constant3/1 -> Matrix Concatenate1/2
  Gain/1 -> Matrix Concatenate1/3
  Constant4/1 -> Sum/2
  Constant1/1 -> Matrix Concatenate/2
  Matrix Concatenate1/1 -> Zero-Order Hold1/1
  Selector1/1 -> Sum/1
  Constant/1 -> Matrix Concatenate/3
  Zero-Order Hold/1 -> Orientation/1
  Zero-Order Hold1/1 -> Position/1
  Selector4/1 -> Gain/1
  Selector3/1 -> Matrix Concatenate1/1
  Pose/1 -> Selector1/1, Selector4/1, Selector3/1

== system MOBATSim/Vehicle Model 10/Vehicle Model - Kinematic 3DOF Single Track ==
  WhlAngF : Inport
  xdotin : Inport  Port=2
  Bicycle Kinematic Model : robotmobilelib/Bicycle Kinematic Model  VehicleInputs=Vehicle Speed & Steering Angle  WheelBase=3  VehicleSpeedRange=[-inf inf]  MaxSteeringAngle=pi/4  InitialState=[Vehicles(Vehicle_id).dynamics.position(1); -Vehicles(Vehicle_id).dynamics.position(3);Vehicles(Vehicle_id).dynamics.orientation(4)]  SimulateUsing=Interpreted execution
      settings: SourceProductBaseCode=RO
  Delay : Delay  DelayLength=1
  Selector3 : Selector  InputPortWidth=3  IndexOptions=Index vector (dialog)  Indices=[1]  OutputSizes=1
  Selector4 : Selector  InputPortWidth=3  IndexOptions=Index vector (dialog)  Indices=[2]  OutputSizes=1
  Sqrt : Sqrt  SaturateOnIntegerOverflow=on
  Square : Math  Operator=square  SaturateOnIntegerOverflow=on
  Square1 : Math  Operator=square  SaturateOnIntegerOverflow=on
  Sum1 : Sum  Inputs=|++
  Pose : Outport
  xdot : Outport  Port=2
  wires:
  WhlAngF/1 -> Bicycle Kinematic Model/2
  xdotin/1 -> Bicycle Kinematic Model/1
  Bicycle Kinematic Model/2 -> Selector3/1, Selector4/1
  Selector3/1 -> Square/1
  Sum1/1 -> Sqrt/1
  Square1/1 -> Sum1/2
  Selector4/1 -> Square1/1
  Sqrt/1 -> Delay/1
  Square/1 -> Sum1/1
  Delay/1 -> xdot/1
  Bicycle Kinematic Model/1 -> Pose/1

== system MOBATSim/Vehicle Model 2/Longitudinal and Lateral Controllers ==
  Speed Reference : Inport
  Inter Vehicular Distance : Inport  Port=2
  Lead Speed : Inport  Port=3
  Driving Mode : Inport  Port=4
  Dist2Stop : Inport  Port=5
  laneChange : Inport  Port=6
  Actual Pose : Inport  Port=7
  Actual Speed : Inport  Port=8
  Lateral Motion Control : Subsystem
  Longitudinal Speed Control : Subsystem
  Longitudinal Acceleration Cmd : Outport
  Reference Steering Angle : Outport  Port=2
  wires:
  Driving Mode/1 -> Longitudinal Speed Control/4(Driving Mode)
  Inter Vehicular Distance/1 -> Longitudinal Speed Control/2(Inter Vehicular Distance)
  Speed Reference/1 -> Longitudinal Speed Control/1(Speed Reference)
  Lead Speed/1 -> Longitudinal Speed Control/3(Lead Speed)
  Dist2Stop/1 -> Longitudinal Speed Control/5(Dist2Stop)
  Lateral Motion Control/1(Reference Steering Angle) -> Reference Steering Angle/1
  Actual Speed/1 -> Longitudinal Speed Control/6(Actual Speed), Lateral Motion Control/1(Speed)
  laneChange/1 -> Lateral Motion Control/3(laneChange)
  Actual Pose/1 -> Lateral Motion Control/2(Pose)
  Longitudinal Speed Control/1(Longitduinal Acceleration Command) -> Longitudinal Acceleration Cmd/1

== system MOBATSim/Vehicle Model 2/Safety Filter ==
  note: Longitudinal
  Reference Acceleration : Inport
  Reference Steering Angle : Inport  Port=2
  Acceleration to Speed : Integrator  LimitOutput=on  LowerSaturationLimit=0
  MATLAB System : MATLABSystem  System=VehicleSafetyFilter  Vehicle_id=Vehicle_id  SimulateUsing=Interpreted execution
      mask Type: VehicleSafetyFilter
      mask Display:
      | disp('VehicleSafetyFilter');
      | port_label('input',1,'Acc');
      | port_label('input',2,'Steering');
      | port_label('output',1,'Acc');
      | port_label('output',2,'Stop');
      | port_label('output',3,'Steering');
  Product : Product
  Signal Specification : SignalSpecification  Dimensions=1
  Stop Check : simulink/Logic and Bit Operations/Compare To Constant  relop=~=  const=1  OutDataTypeStr=uint8
  Zero-Order Hold : ZeroOrderHold  SampleTime=Sim_Ts
  Speed_input : Outport
  Steering Angle Cmd : Outport  Port=2
  wires:
  Acceleration to Speed/1 -> Signal Specification/1
  Stop Check/1 -> Product/2
  Signal Specification/1 -> Zero-Order Hold/1
  Reference Acceleration/1 -> MATLAB System/1
  Zero-Order Hold/1 -> Product/1
  Product/1 -> Speed_input/1
  MATLAB System/1 -> Acceleration to Speed/1
  Reference Steering Angle/1 -> MATLAB System/2
  MATLAB System/3 -> Steering Angle Cmd/1
  MATLAB System/2 -> Stop Check/1

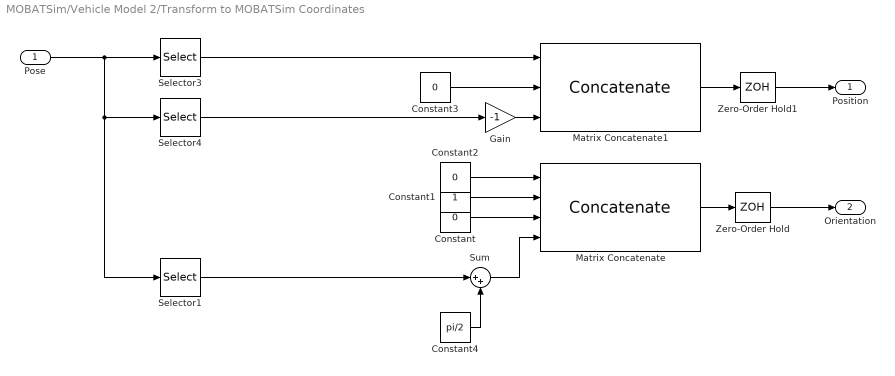
== system MOBATSim/Vehicle Model 2/Transform to MOBATSim Coordinates ==
  Pose : Inport
  Constant : Constant  Value=0
  Constant1 : Constant
  Constant2 : Constant  Value=0
  Constant3 : Constant  Value=0
  Constant4 : Constant  Value=pi/2
  Gain : Gain  Gain=-1
  Matrix Concatenate : Concatenate  NumInputs=4  ConcatenateDimension=2
  Matrix Concatenate1 : Concatenate  NumInputs=3  ConcatenateDimension=2
  Selector1 : Selector  InputPortWidth=3  IndexOptions=Index vector (dialog)  Indices=[3]  OutputSizes=1
  Selector3 : Selector  InputPortWidth=3  IndexOptions=Index vector (dialog)  Indices=[1]  OutputSizes=1
  Selector4 : Selector  InputPortWidth=3  IndexOptions=Index vector (dialog)  Indices=[2]  OutputSizes=1
  Sum : Sum  Inputs=|++
  Zero-Order Hold : ZeroOrderHold  SampleTime=Sim_Ts
  Zero-Order Hold1 : ZeroOrderHold  SampleTime=Sim_Ts
  Position : Outport
  Orientation : Outport  Port=2
  wires:
  Sum/1 -> Matrix Concatenate/4
  Constant2/1 -> Matrix Concatenate/1
  Matrix Concatenate/1 -> Zero-Order Hold/1
  Constant3/1 -> Matrix Concatenate1/2
  Gain/1 -> Matrix Concatenate1/3
  Constant4/1 -> Sum/2
  Constant1/1 -> Matrix Concatenate/2
  Matrix Concatenate1/1 -> Zero-Order Hold1/1
  Selector1/1 -> Sum/1
  Constant/1 -> Matrix Concatenate/3
  Zero-Order Hold/1 -> Orientation/1
  Zero-Order Hold1/1 -> Position/1
  Selector4/1 -> Gain/1
  Selector3/1 -> Matrix Concatenate1/1
  Pose/1 -> Selector1/1, Selector4/1, Selector3/1

== system MOBATSim/Vehicle Model 2/Vehicle Model - Kinematic 3DOF Single Track ==
  Longitudinal Speed : Inport
  Steering Angle : Inport  Port=2
  Bicycle Kinematic Model : robotmobilelib/Bicycle Kinematic Model  VehicleInputs=Vehicle Speed & Steering Angle  WheelBase=3  VehicleSpeedRange=[-inf inf]  MaxSteeringAngle=pi/4  InitialState=[Vehicles(Vehicle_id).dynamics.position(1); -Vehicles(Vehicle_id).dynamics.position(3);Vehicles(Vehicle_id).dynamics.orientation(4)]  SimulateUsing=Interpreted execution
      settings: SourceProductBaseCode=RO
  Delay : Delay  DelayLength=1
  Selector3 : Selector  InputPortWidth=3  IndexOptions=Index vector (dialog)  Indices=[1]  OutputSizes=1
  Selector4 : Selector  InputPortWidth=3  IndexOptions=Index vector (dialog)  Indices=[2]  OutputSizes=1
  Sqrt : Sqrt  SaturateOnIntegerOverflow=on
  Square : Math  Operator=square  SaturateOnIntegerOverflow=on
  Square1 : Math  Operator=square  SaturateOnIntegerOverflow=on
  Sum1 : Sum  Inputs=|++
  Pose : Outport
  Speed : Outport  Port=2
  wires:
  Delay/1 -> Speed/1
  Bicycle Kinematic Model/1 -> Pose/1
  Selector4/1 -> Square1/1
  Longitudinal Speed/1 -> Bicycle Kinematic Model/1
  Steering Angle/1 -> Bicycle Kinematic Model/2
  Sum1/1 -> Sqrt/1
  Sqrt/1 -> Delay/1
  Square/1 -> Sum1/1
  Square1/1 -> Sum1/2
  Selector3/1 -> Square/1
  Bicycle Kinematic Model/2 -> Selector4/1, Selector3/1

== system MOBATSim/Vehicle Model 3/Longitudinal and Lateral Controllers ==
  Speed Reference : Inport
  Inter Vehicular Distance : Inport  Port=2
  Lead Speed : Inport  Port=3
  drivingMode : Inport  Port=4
  Dist2Stop : Inport  Port=5
  laneChange : Inport  Port=6
  Actual Speed : Inport  Port=7
  Actual Pose : Inport  Port=8
  Lateral Control : Subsystem
  Longitudinal Speed Control : Subsystem
  ref Acc : Outport
  ref Steering : Outport  Port=2
  wires:
  laneChange/1 -> Lateral Control/3(laneChange)
  Lateral Control/1(SteerCmd_Stanley) -> ref Steering/1
  Actual Speed/1 -> Longitudinal Speed Control/6(Actual Speed), Lateral Control/1(actualSpeed)
  drivingMode/1 -> Longitudinal Speed Control/4(Driving Mode)
  Longitudinal Speed Control/1(Longitduinal Acceleration Command) -> ref Acc/1
  Dist2Stop/1 -> Longitudinal Speed Control/5(Dist2Stop)
  Inter Vehicular Distance/1 -> Longitudinal Speed Control/2(Inter Vehicular Distance)
  Lead Speed/1 -> Longitudinal Speed Control/3(Lead Speed)
  Speed Reference/1 -> Longitudinal Speed Control/1(Speed Reference)
  Actual Pose/1 -> Lateral Control/2(actualPose)
